simulink model "PCT_model"  (R2021a)
settings: Solver=VariableStepAuto  StartTime=0.0  StopTime=10.0  RelTol=1e-3
undefined symbols (not defined in the file or in its folder): Disk, Floor, to, wo, X, Y, Z
libraries: sm_lib x66, nesl_utility x16, pid_lib x3, Contact_Forces_Lib x1, simulink x1, Parts_Lib x1, Multibody_Multiphysics_Lib x1
(part 3 of 3)

== matlab function PCT_model/MATLAB Function1 ==
  settings: updateMethod=DISCRETE
  data: a output; a input; u1 input; u2 input; xy1 input; xy2 input; y1 input; fvel output; y2 input; bh input; lvel output; angley3 input; fvel input; lvel input; v input; ld input; ld output; v output; y1 output; y2 output; dt input
function [a,fvel,lvel,ld,v,y1,y2] = find_yvels(a,u1,u2,xy1,xy2,y1,y2,bh,angley3,fvel,lvel,v,ld,dt)
            %% initial y1 y2 impulses
            %y1 y2 are t-1 values, xy1, xy2 are t(current values)
            
            %a mimics t, time counter
            if a ==0
                y1=u1;
                y2=u2;
                a=1;
            elseif a==1
                y1=y1;
                y2=y2;
                a=2;
                if fvel==0 %initial values for fvel, lvel
                    fvel=xy1-y1;
                end
                if lvel==0
                    lvel=xy2-y2;
                end
            else
                %
            end
            
            if a>=2
                %%
                delay = zeros(3,5);

                %y1,y2, angley(t-1)
                ld_temp = bh+(y1); %*cos(angley1(t)) %was 5-minus
                % v is retina2, relate ball and actuator 2
                %v(t) = len-bh(t)-(5-y2(t-1)*sin(angley3(t-1)));
                v_temp = bh+(y2*cos(angley3)); %was sin, but sin(pi/2)=0., was 5-y2*

                p1 = v_temp-v;
                p2 = ld_temp-ld;
                v=v_temp;
                ld=ld_temp;

                %% Solve for actuators
                % Matlab Cannot Iterate over 0 index, hence 1-4 with Minus 1
                for j = 1:1:4
                    delay(2,j+1) = delay(2,j);
                    delay(3,j+1) = delay(3,j);
                end

                %%
                    x = 0; x1 = 0; x2 = 0; x3 = 0; x4 = 0; nu = 0; d = zeros(1,800);
                    constant = 5.0; max = 0; 
                    xmin=0; xmax=1; n=1;
                    rand_x = xmin+rand(1,n)*(xmax-xmin);

                    for i = 1:1:400
                        rand_x = rand_num();
                        x =  0.5 - rand_x;
                        x1 = x1+(x-x1)/constant;
                        x2 = x2+(x1-x2)/constant;
                        x3 = x3+(x2-x3)/constant;
                        x4 = x4+(x3-x4)/constant;
                    end

                    for i = 1:1:800
                        rand_x = rand_num();
                        x = 0.5 - rand_x;
                        x1 = x1+(x-x1)/constant;
                        x2 = x2+(x1-x2)/constant;
                        x3 = x3+(x2-x3)/constant;
                        x4 = x4+(x3-x4)/constant;
                        d(i) = (10000*x4);
                    end

                    for i = 1:1:800
                        if (d(i) > max)
                            max = abs(d(i));
                        end
                    end

                    for i = 1:1:800
                        d(i)  = d(i)/(max) * 100.0;
                    end
                %%
                noisy = d;

                delay(2,1) = p1 + noisy(1)/30000.0; %delays relat ld & v to velocities later. 
                delay(3,1) = p2 + noisy(1)/30000.0;

                fgain=300;lgain=300;fslow=500;lslow=500;
                ref1= 0.0185; ref2 = 0.0185;
                %fvel(t) = fvel(t-1) + (fgain * (ref1-delay(1,1))-fvel(t-1))/fslow; %actuator 1 velocity -> relate to ld
                %lvel(t) = lvel(t-1) + (lgain * (ref2-delay(1,1))-lvel(t-1))/lslow; %actuator 2 verlocity -> relate to v           

                fvel = fvel + (fgain * (ref1-delay(2,1))-fvel)/fslow; 
                lvel = lvel + (lgain * (ref2-delay(3,1))-lvel)/lslow; %was minus

                y1 = y1 - fvel*dt; %was plus, use adjusted speed? t+1? 
                y2 = y2 - lvel*dt;
            end
end

== matlab function PCT_model/MATLAB Function ==
  data: y1 input; A output; y2 input; len input
function A = concat_A(y1,y2,len)
 A=[len y1 y2];
end

== matlab function PCT_model/MATLAB Function2 ==
  data: cv input; dt input; cv output; g input; angley1 input; y1 input; y2 input
function cv = fcn(cv,dt,g,angley1,y1,y2)

            a_mult_t=dt*g*cos(angley1);
        %
            if y1>y2
            cv = cv+a_mult_t*sin(angley1);
        else %y2>y1
            cv = cv+a_mult_t*cos(angley1-pi/2);
        end
            %}
         %cv = cv+a_mult_t*sin(angley1);
end

== matlab function PCT_model/MATLAB Function3 ==
  data: y1 input; angley1 output; y2 input; angley2 output; angley3 output; x1 input; x2 input
    function [angley1,angley2,angley3] = find_angleys(y1,y2,x1,x2)


    if y1>y2
        %use value set 1
        angley1=x1(1)+pi/2;  %mtrig manipulation to put in right quadrant
        angley2=0.5*pi-angley1; %internal angles of a right-angle-triangle
        angley3=x1(2);
    else %y2>=y1
        %use value set 2
        angley1=pi/2-x2(1);  %mtrig manipulation to put in right quadrant???
        angley2= -(0.5*pi-(pi-angley1)); %internal angles of a right-angle-triangle
        angley3=x2(2);
    end
        
end
